simulink model "Flight_Model_2021a_10_12_2021"  (R2021a)
settings: Solver=VariableStepAuto  StartTime=0.0  StopTime=100  RelTol=1e-3
model workspace (MAT data in the model file):
  bodyLength = 5
  brakesCd = 1
  brakesOn = 1
  dryCG = 1.9
  dryMass = 23
  finArea = 0.2
  finChordAngle = 0.5236
  finSpan = 0.4
  fullBrakesOn = 0
  gravity = 9.8067
  noseLength = 0.5
  propMass = 7.183
  refArea = 0.0182
  rocketCP = 1
  rocketDiam = 0.197
  targetAlt = 3048
  thrust = [0; 2638.366; 2528.97; 3063.078; 2426.009; 2548.275; 2599.755; 2554.71; 2644.801; 2638.366; 2561.145; 2606.19; 2638.366; 2638.366; 2580.45; 2496.795; 2335.919; 2213.653; 2129.998; 1653.805; 888.035; 630.634; 450.453; 289.577; 135.136; 25.74; 0]
  time = [0; 0.045; 0.067; 0.084; 0.124; 0.186; 0.231; 0.298; 0.371; 0.534; 0.979; 1.142; 2.002; 2.289; 2.761; 3.121; 3.436; 3.678; 3.79; 4.004; 4.415; 4.538; 4.656; 4.82; 5.005; 5.219; 5.371]
  totalImpulse = 10831
  vehicleCd = 0.8
  wetCG = 2.1
  wetMass = 30
libraries: aerolibasang x4, aerolibbdyn x2, aerolibwind2 x2, aerolibatmos2 x1, shared6dof x1
settings Model: OrderedModelArguments=off  Creator=alhus  LastModifiedBy=alhus

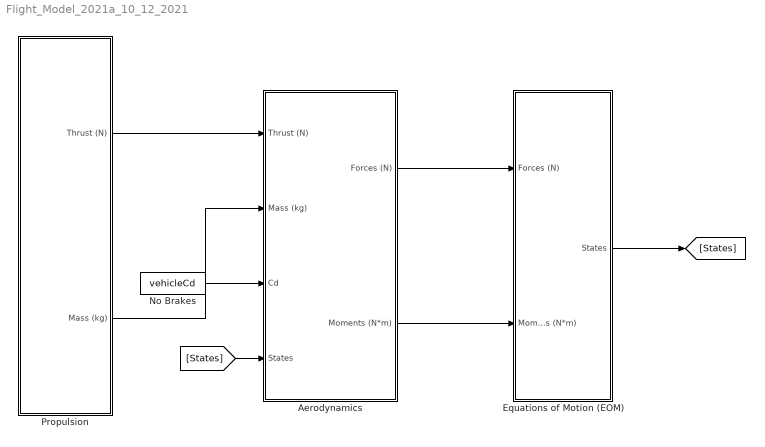
== system Flight_Model_2021a_10_12_2021 ==
  Aerodynamics : Subsystem
  Equations of Motion (EOM) : Subsystem
  No Brakes : Constant  Value=vehicleCd
  Propulsion : Subsystem
  wires:
  Propulsion/1(Thrust (N)) -> Aerodynamics/1(Thrust (N))
  Propulsion/2(Mass (kg)) -> Aerodynamics/2(Mass (kg))
  [States] -> Aerodynamics/4(States)
  No Brakes/1 -> Aerodynamics/3(Cd)
  Aerodynamics/2(Moments (N*m)) -> Equations of Motion (EOM)/2(Moments (N*m))
  Aerodynamics/1(Forces (N)) -> Equations of Motion (EOM)/1(Forces (N))
  Equations of Motion (EOM)/1(States) -> [States]

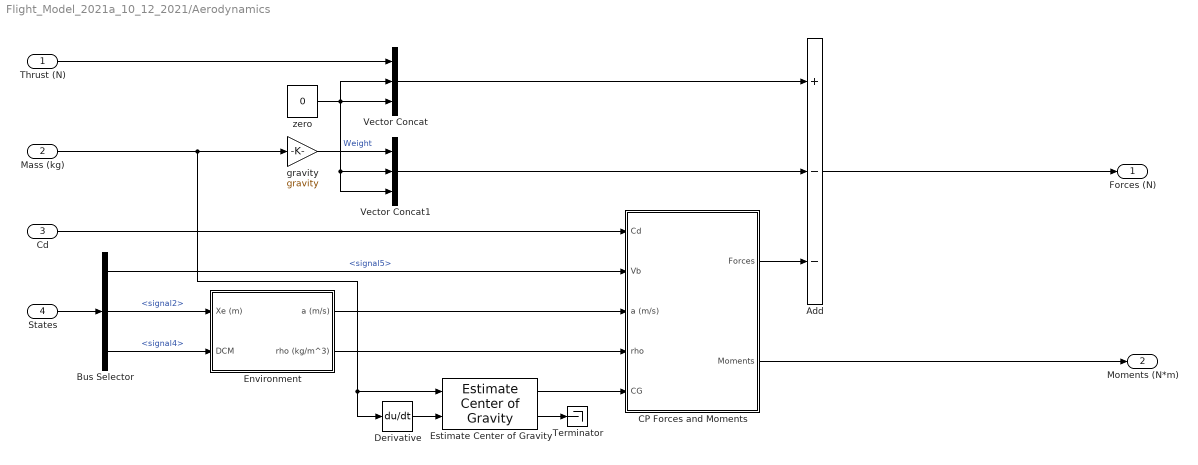
== system Flight_Model_2021a_10_12_2021/Aerodynamics ==
  Thrust (N) : Inport
  Mass (kg) : Inport  Port=2
  Cd : Inport  Port=3
  States : Inport  Port=4
  Add : Sum  Inputs=+--
  Bus Selector : BusSelector  OutputSignals=signal5,signal2,signal4
  CP Forces and Moments : Subsystem
  Derivative : Derivative
  Environment : Subsystem
  Estimate Center of Gravity : aerolibbdyn/Estimate Center of Gravity  fmass=wetMass  emass=dryMass  fcg=[wetCG 0 0]'  ecg=[dryCG 0 0]'
      settings: SourceProductBaseCode=AE
  Terminator : Terminator
  Vector Concat : Concatenate  NumInputs=3
  Vector Concat1 : Concatenate  NumInputs=3
  gravity : Gain  Gain=gravity
  "zero " : Constant  Value=0
  Forces (N) : Outport
  Moments (N*m) : Outport  Port=2
  wires:
  Mass (kg)/1 -> Derivative/1, Estimate Center of Gravity/1, gravity/1
  Derivative/1 -> Estimate Center of Gravity/2
  Estimate Center of Gravity/2 -> Terminator/1
  Estimate Center of Gravity/1 -> CP Forces and Moments/5(CG)
  Cd/1 -> CP Forces and Moments/1(Cd)
  Environment/2(rho (kg/m^3)) -> CP Forces and Moments/4(rho)
  CP Forces and Moments/2(Moments) -> Moments (N*m)/1
  States/1 -> Bus Selector/1
  Environment/1(a (m/s)) -> CP Forces and Moments/3(a (m/s))
  Bus Selector/1 -> CP Forces and Moments/2(Vb)  "<signal5>"
  Bus Selector/2 -> Environment/1(Xe (m))  "<signal2>"
  Bus Selector/3 -> Environment/2(DCM)  "<signal4>"
  "zero "/1 -> Vector Concat/2, Vector Concat/3, Vector Concat1/2, Vector Concat1/3
  Thrust (N)/1 -> Vector Concat/1
  Vector Concat/1 -> Add/1
  Vector Concat1/1 -> Add/2
  gravity/1 -> Vector Concat1/1  "Weight"
  CP Forces and Moments/1(Forces) -> Add/3
  Add/1 -> Forces (N)/1

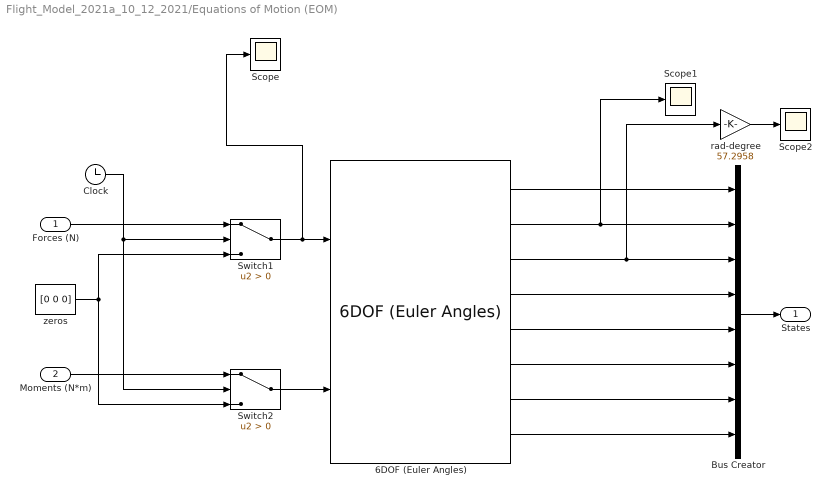
== system Flight_Model_2021a_10_12_2021/Equations of Motion (EOM) ==
  Forces (N) : Inport
  Moments (N*m) : Inport  Port=2
  6DOF (Euler Angles) : shared6dof/6DOF (Euler Angles)  units=Metric (MKS)  mtype=Fixed  rep=Euler Angles  xme_0=[0 0 0]  Vm_0=[0 0 0]  eul_0=[0 0 0]  pm_0=[0, 0, 0]  mass_0=30  mass_e=0.5  mass_f=2.0  inertia=eye(3)  inertia_e=eye(3)  inertia_f=2*eye(3)  k_quat=1.0  vre_flag=on  abi_flag=off  aMode=aMode  xme_statename=''  Vm_statename=''  eul_statename=''  quat_statename=''  pm_statename=''  mass_statename=''
      settings: SourceProductBaseCode=AE,PW,MT,UV,VE,VP
  Bus Creator : BusCreator  Inputs=8
  Clock : Clock
  Scope : Scope
  Scope1 : Scope
  Scope2 : Scope
  Switch1 : Switch  Criteria=u2 > Threshold
  Switch2 : Switch  Criteria=u2 > Threshold
  rad-degree : Gain  Gain=57.2958
  "zeros " : Constant  Value=[0 0 0]
  States : Outport
  wires:
  "zeros "/1 -> Switch2/3, Switch1/3
  Switch2/1 -> 6DOF (Euler Angles)/2
  Forces (N)/1 -> Switch1/1
  6DOF (Euler Angles)/1 -> Bus Creator/1
  6DOF (Euler Angles)/4 -> Bus Creator/4
  6DOF (Euler Angles)/7 -> Bus Creator/7
  Clock/1 -> Switch2/2, Switch1/2
  6DOF (Euler Angles)/8 -> Bus Creator/8
  6DOF (Euler Angles)/3 -> rad-degree/1, Bus Creator/3
  6DOF (Euler Angles)/6 -> Bus Creator/6
  6DOF (Euler Angles)/2 -> Scope1/1, Bus Creator/2
  Switch1/1 -> Scope/1, 6DOF (Euler Angles)/1
  6DOF (Euler Angles)/5 -> Bus Creator/5
  Bus Creator/1 -> States/1
  Moments (N*m)/1 -> Switch2/1
  rad-degree/1 -> Scope2/1

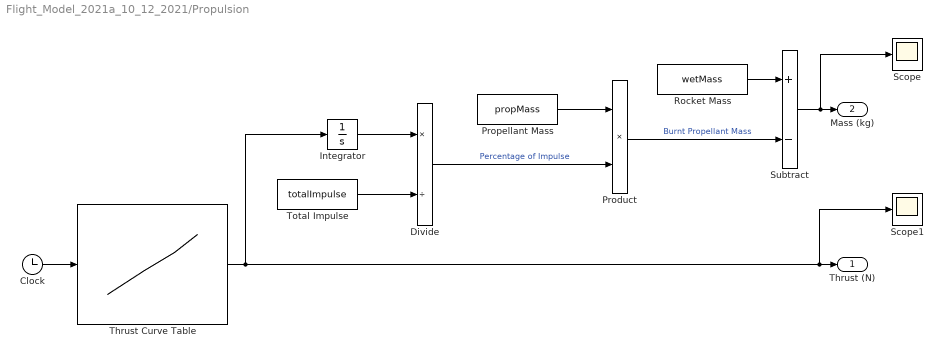
== system Flight_Model_2021a_10_12_2021/Propulsion ==
  Clock : Clock
  Divide : Product  Inputs=*/
  Integrator : Integrator
  Product : Product
  Propellant Mass : Constant  Value=propMass
  Rocket Mass : Constant  Value=wetMass
  Scope : Scope
  Scope1 : Scope
  Subtract : Sum  Inputs=+-
  Thrust Curve Table : Lookup_n-D  NumberOfTableDimensions=1  BreakpointsForDimension1=time  Table=thrust  ExtrapMethod=Clip  InternalRulePriority=Speed  RndMeth=Simplest  InputSameDT=on
  Total Impulse : Constant  Value=totalImpulse
  Thrust (N) : Outport
  Mass (kg) : Outport  Port=2
  wires:
  Total Impulse/1 -> Divide/2
  Integrator/1 -> Divide/1
  Clock/1 -> Thrust Curve Table/1
  Propellant Mass/1 -> Product/1
  Product/1 -> Subtract/2  "Burnt Propellant Mass"
  Rocket Mass/1 -> Subtract/1
  Subtract/1 -> Scope/1, Mass (kg)/1
  Thrust Curve Table/1 -> Scope1/1, Thrust (N)/1, Integrator/1
  Divide/1 -> Product/2  "Percentage of Impulse"

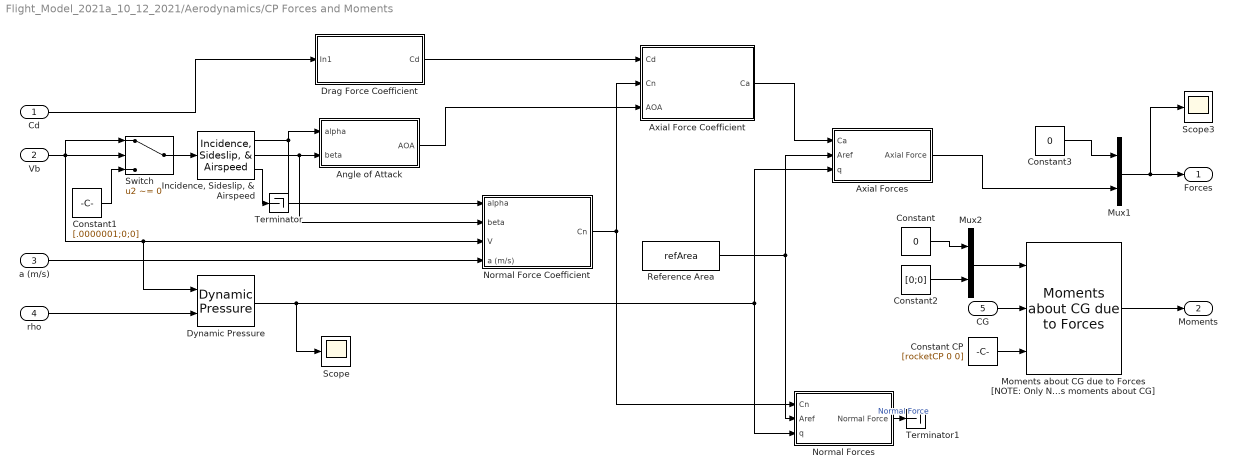
== system Flight_Model_2021a_10_12_2021/Aerodynamics/CP Forces and Moments ==
  Cd : Inport
  Vb : Inport  Port=2
  a (m/s) : Inport  Port=3
  rho : Inport  Port=4
  CG : Inport  Port=5
  Angle of Attack : Subsystem
  Axial Force Coefficient : Subsystem
  Axial Forces : Subsystem
  Constant : Constant  Value=0
  Constant CP : Constant  Value=[rocketCP 0 0]
  Constant1 : Constant  Value=[.0000001;0;0]  VectorParams1D=off
  Constant2 : Constant  Value=[0;0]  VectorParams1D=off
  Constant3 : Constant  Value=0
  Drag Force Coefficient : Subsystem
  Dynamic Pressure : aerolibasang/Dynamic Pressure
  "Incidence, Sideslip, & Airspeed" : aerolibasang/Incidence, Sideslip, & Airspeed
  Moments about CG due to Forces [NOTE: Only Normal Force applys moments about CG] : aerolibbdyn/Moments about CG  due to Forces
      settings: SourceProductBaseCode=AE
  Mux1 : Mux  Inputs=2
  Mux2 : Mux  Inputs=2
  Normal Force Coefficient : Subsystem
  Normal Forces : Subsystem
  Reference Area : Constant  Value=refArea
  Scope : Scope
  Scope3 : Scope
  Switch : Switch  Criteria=u2 ~= 0
  Terminator : Terminator
  Terminator1 : Terminator
  Forces : Outport
  Moments : Outport  Port=2
  wires:
  CG/1 -> Moments about CG due to Forces [NOTE: Only Normal Force applys moments about CG]/2
  Drag Force Coefficient/1(Cd) -> Axial Force Coefficient/1(Cd)
  rho/1 -> Dynamic Pressure/2
  a (m/s)/1 -> Normal Force Coefficient/4(a (m/s))
  Dynamic Pressure/1 -> Scope/1, Normal Forces/3("q "), Axial Forces/3("q ")
  Angle of Attack/1(AOA) -> Axial Force Coefficient/3(AOA)
  Cd/1 -> Drag Force Coefficient/1(In1)
  Reference Area/1 -> Normal Forces/2(Aref), Axial Forces/2(Aref)
  Constant CP/1 -> Moments about CG due to Forces [NOTE: Only Normal Force applys moments about CG]/3
  Moments about CG due to Forces [NOTE: Only Normal Force applys moments about CG]/1 -> Moments/1
  "Incidence, Sideslip, & Airspeed"/2 -> Normal Force Coefficient/2(beta), Angle of Attack/2(beta)
  "Incidence, Sideslip, & Airspeed"/3 -> Terminator/1
  Normal Force Coefficient/1(Cn) -> Axial Force Coefficient/2(Cn), Normal Forces/1(Cn)
  "Incidence, Sideslip, & Airspeed"/1 -> Angle of Attack/1(alpha), Normal Force Coefficient/1(alpha)
  Axial Force Coefficient/1(Ca) -> Axial Forces/1(Ca)
  Mux1/1 -> Scope3/1, Forces/1
  Constant2/1 -> Mux2/2
  Mux2/1 -> Moments about CG due to Forces [NOTE: Only Normal Force applys moments about CG]/1
  Normal Forces/1(Normal Force) -> Terminator1/1  "Normal Force"
  Constant/1 -> Mux2/1
  Axial Forces/1(Axial Force) -> Mux1/2
  Constant3/1 -> Mux1/1
  Vb/1 -> Switch/1, Switch/2, Normal Force Coefficient/3(V), Dynamic Pressure/1
  Switch/1 -> "Incidence, Sideslip, & Airspeed"/1
  Constant1/1 -> Switch/3

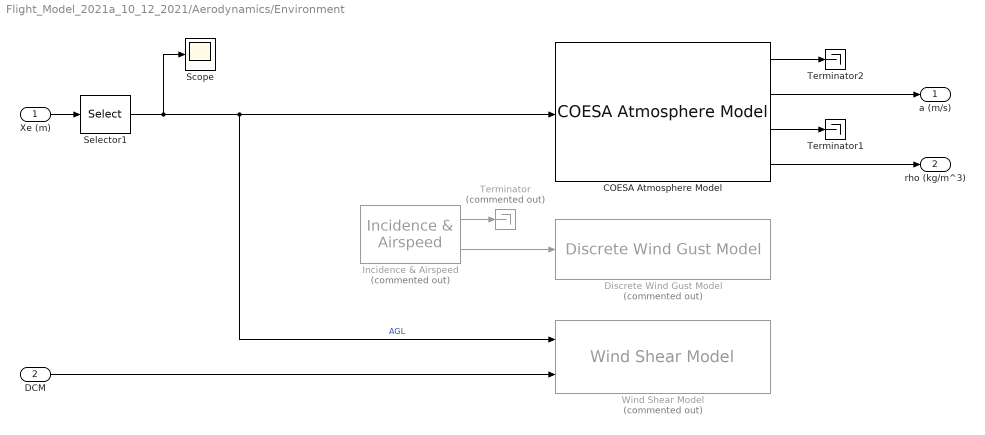
== system Flight_Model_2021a_10_12_2021/Aerodynamics/Environment ==
  Xe (m) : Inport
  DCM : Inport  Port=2
  COESA Atmosphere Model : aerolibatmos2/COESA Atmosphere Model  units=Metric (MKS)  spec=1976 COESA-extended U.S. Standard Atmosphere  model=Profile  profile_var=High temperature  profile_percent=1%  profile_alt=5 km (16404 ft)  envelope_var=High temperature  envelope_percent=1%  action=Warning
  Discrete Wind Gust Model : aerolibwind2/Discrete Wind Gust Model  Commented=on  units=Metric (MKS)  Gx=on  Gy=on  Gz=on  t_0=5  d_m=[120 120 80]  v_m=[3.5 3.5 3.0]
  Incidence & Airspeed : aerolibasang/Incidence  & Airspeed  Commented=on
      settings: SourceProductBaseCode=AE
  Scope : Scope
  Selector1 : Selector  InputPortWidth=3  IndexOptions=Index vector (dialog)  Indices=3  OutputSizes=1
  Terminator : Terminator  Commented=on
  Terminator1 : Terminator
  Terminator2 : Terminator
  Wind Shear Model : aerolibwind2/Wind Shear Model  Commented=on  units=Metric (MKS)  phase=Category C - Terminal Flight Phase  W_20=15  Wdeg=0
  a (m/s) : Outport
  rho (kg/m^3) : Outport  Port=2
  wires:
  Incidence & Airspeed/2 -> Discrete Wind Gust Model/1
  Incidence & Airspeed/1 -> Terminator/1
  Xe (m)/1 -> Selector1/1
  DCM/1 -> Wind Shear Model/2
  Selector1/1 -> Wind Shear Model/1, COESA Atmosphere Model/1, Scope/1  "AGL"
  COESA Atmosphere Model/2 -> a (m/s)/1
  COESA Atmosphere Model/4 -> rho (kg/m^3)/1
  COESA Atmosphere Model/1 -> Terminator2/1
  COESA Atmosphere Model/3 -> Terminator1/1

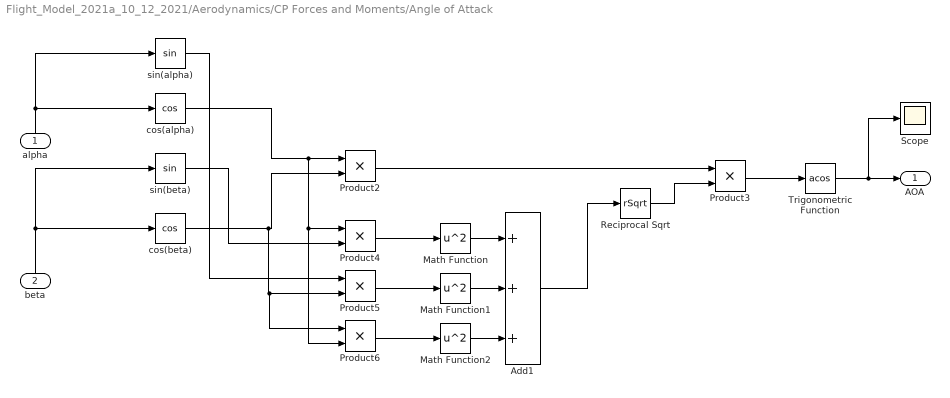
== system Flight_Model_2021a_10_12_2021/Aerodynamics/CP Forces and Moments/Angle of Attack ==
  alpha : Inport
  beta : Inport  Port=2
  Add1 : Sum  Inputs=+++
  Math Function : Math  Operator=square  SignedPower=on  SaturateOnIntegerOverflow=on
  Math Function1 : Math  Operator=square  SignedPower=on  SaturateOnIntegerOverflow=on
  Math Function2 : Math  Operator=square  SignedPower=on  SaturateOnIntegerOverflow=on
  Product{2..6} (5 alike) : Product
  Reciprocal Sqrt : Sqrt  Operator=rSqrt  SaturateOnIntegerOverflow=on
  Scope : Scope
  Trigonometric Function : Trigonometry  Operator=acos
  cos(alpha) : Trigonometry  Operator=cos
  cos(beta) : Trigonometry  Operator=cos
  sin(alpha) : Trigonometry
  sin(beta) : Trigonometry
  AOA : Outport
  wires:
  Product3/1 -> Trigonometric Function/1
  Math Function2/1 -> Add1/3
  Product5/1 -> Math Function1/1
  Product6/1 -> Math Function2/1
  alpha/1 -> cos(alpha)/1, sin(alpha)/1
  cos(alpha)/1 -> Product6/2, Product4/1, Product2/1
  beta/1 -> cos(beta)/1, sin(beta)/1
  cos(beta)/1 -> Product6/1, Product5/2, Product2/2
  Reciprocal Sqrt/1 -> Product3/2
  Math Function/1 -> Add1/1
  Math Function1/1 -> Add1/2
  sin(beta)/1 -> Product4/2
  Add1/1 -> Reciprocal Sqrt/1
  sin(alpha)/1 -> Product5/1
  Product2/1 -> Product3/1
  Product4/1 -> Math Function/1
  Trigonometric Function/1 -> Scope/1, AOA/1

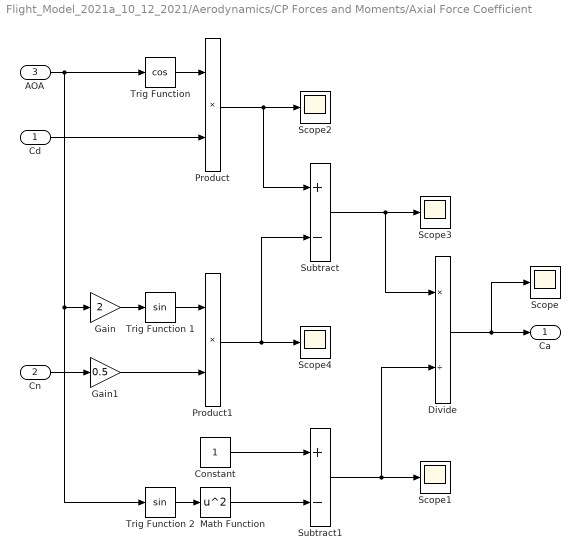
== system Flight_Model_2021a_10_12_2021/Aerodynamics/CP Forces and Moments/Axial Force Coefficient ==
  Cd : Inport
  Cn : Inport  Port=2
  AOA : Inport  Port=3
  Constant : Constant
  Divide : Product  Inputs=*/
  Gain : Gain  Gain=2
  Gain1 : Gain  Gain=0.5
  Math Function : Math  Operator=square  SignedPower=on  SaturateOnIntegerOverflow=on
  Product : Product
  Product1 : Product
  Scope{,1..4} (5 alike) : Scope
  Subtract : Sum  Inputs=+-
  Subtract1 : Sum  Inputs=+-
  Trig Function : Trigonometry  Operator=cos
  Trig Function 1 : Trigonometry
  Trig Function 2 : Trigonometry
  Ca : Outport
  wires:
  AOA/1 -> Trig Function/1, Trig Function 2/1, Gain/1
  Cd/1 -> Product/2
  Trig Function/1 -> Product/1
  Gain/1 -> Trig Function 1/1
  Trig Function 1/1 -> Product1/1
  Gain1/1 -> Product1/2
  Cn/1 -> Gain1/1
  Product1/1 -> Scope4/1, Subtract/2
  Divide/1 -> Scope/1, Ca/1
  Trig Function 2/1 -> Math Function/1
  Math Function/1 -> Subtract1/2
  Constant/1 -> Subtract1/1
  Subtract/1 -> Scope3/1, Divide/1
  Subtract1/1 -> Scope1/1, Divide/2
  Product/1 -> Scope2/1, Subtract/1

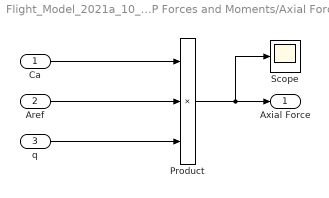
== system Flight_Model_2021a_10_12_2021/Aerodynamics/CP Forces and Moments/Axial Forces ==
  Ca : Inport
  Aref : Inport  Port=2
  "q " : Inport  Port=3
  Product : Product  Inputs=3
  Scope : Scope
  Axial Force : Outport
  wires:
  Ca/1 -> Product/1
  Aref/1 -> Product/2
  Product/1 -> Axial Force/1, Scope/1
  "q "/1 -> Product/3

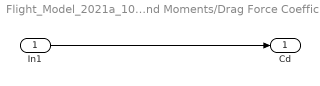
== system Flight_Model_2021a_10_12_2021/Aerodynamics/CP Forces and Moments/Drag Force Coefficient ==
  In1 : Inport
  Cd : Outport
  wires:
  In1/1 -> Cd/1

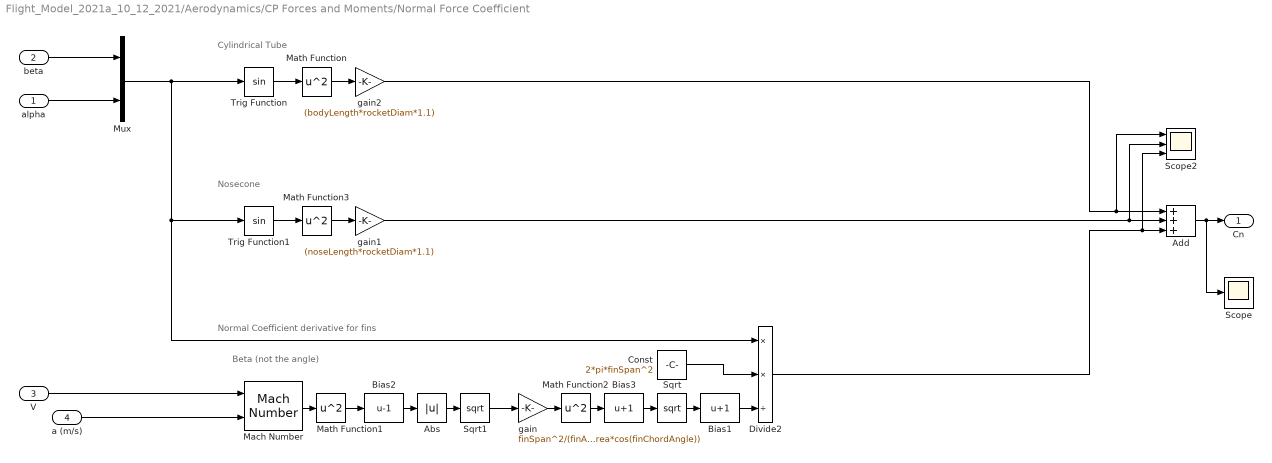
== system Flight_Model_2021a_10_12_2021/Aerodynamics/CP Forces and Moments/Normal Force Coefficient ==
  note: Cylindrical Tube
  note: Normal Coefficient derivative for fins
  note: Beta (not the angle)
  note: Nosecone
  alpha : Inport
  beta : Inport  Port=2
  V : Inport  Port=3
  a (m/s) : Inport  Port=4
  Abs : Abs
  Add : Sum  Inputs=+++
  Bias1 : Bias  Bias=1
  Bias2 : Bias  Bias=-1
  Bias3 : Bias  Bias=1
  Const : Constant  Value=2*pi*finSpan^2
  Divide2 : Product  Inputs=**/
  Mach Number : aerolibasang/Mach Number
      settings: SourceProductBaseCode=AE
  Math Function{,1..3} (4 alike) : Math  Operator=square  SignedPower=on  SaturateOnIntegerOverflow=on
  Mux : Mux  Inputs=2
  Scope : Scope
  Scope2 : Scope  NumInputPorts=3
  Sqrt : Sqrt  SaturateOnIntegerOverflow=on
  Sqrt1 : Sqrt  SaturateOnIntegerOverflow=on
  Trig Function : Trigonometry
  Trig Function1 : Trigonometry
  gain : Gain  Gain=finSpan^2/(finArea*cos(finChordAngle))
  gain1 : Gain  Gain=(noseLength*rocketDiam*1.1)
  gain2 : Gain  Gain=(bodyLength*rocketDiam*1.1)
  Cn : Outport
  wires:
  Trig Function/1 -> Math Function/1
  Sqrt1/1 -> gain/1
  Math Function2/1 -> Bias3/1
  Sqrt/1 -> Bias1/1
  Bias3/1 -> Sqrt/1
  gain/1 -> Math Function2/1
  a (m/s)/1 -> Mach Number/2
  Bias1/1 -> Divide2/3
  Math Function/1 -> gain2/1
  Trig Function1/1 -> Math Function3/1
  Math Function3/1 -> gain1/1
  Add/1 -> Scope/1, Cn/1
  V/1 -> Mach Number/1
  Mach Number/1 -> Math Function1/1
  Math Function1/1 -> Bias2/1
  Bias2/1 -> Abs/1
  Abs/1 -> Sqrt1/1
  Const/1 -> Divide2/2
  gain1/1 -> Scope2/2, Add/2
  gain2/1 -> Add/1, Scope2/1
  Divide2/1 -> Add/3, Scope2/3
  beta/1 -> Mux/1
  Mux/1 -> Divide2/1, Trig Function1/1, Trig Function/1
  alpha/1 -> Mux/2

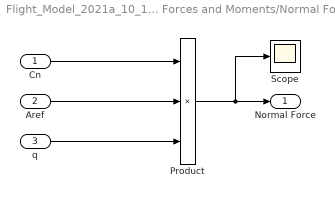
== system Flight_Model_2021a_10_12_2021/Aerodynamics/CP Forces and Moments/Normal Forces ==
  Cn : Inport
  Aref : Inport  Port=2
  "q " : Inport  Port=3
  Product : Product  Inputs=3
  Scope : Scope
  Normal Force : Outport
  wires:
  Cn/1 -> Product/1
  Aref/1 -> Product/2
  Product/1 -> Normal Force/1, Scope/1
  "q "/1 -> Product/3
